simulink model "tutorial40_variant"  (R2025a)
settings: Solver=VariableStepAuto  StartTime=0.0  StopTime=10.0  RelTol=1e-3
settings Model: Creator=xing2  LastModifiedBy=xing2

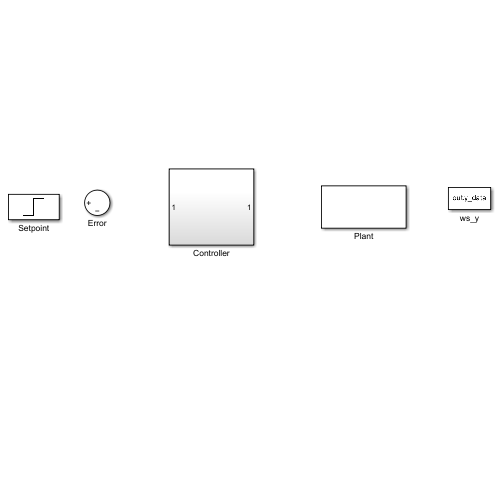
[thumbnail: Simulink's stored preview of the top-level diagram]
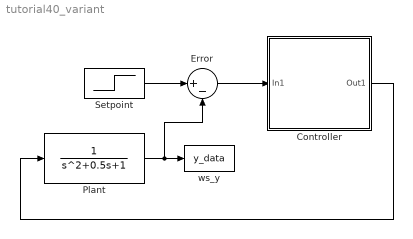
== system tutorial40_variant ==
  Controller : Subsystem  Variant=on
  Error : Sum  Inputs=|+-
  Plant : TransferFcn  Denominator=[1 0.5 1]
  Setpoint : Step  Time=0.5  SampleTime=0
  ws_y : ToWorkspace  VariableName=y_data  SaveFormat=Timeseries  SampleTime=-1
  wires:
  Setpoint/1 -> Error/1
  Plant/1 -> Error/2, ws_y/1
  Error/1 -> Controller/1(In1)
  Controller/1(Out1) -> Plant/1

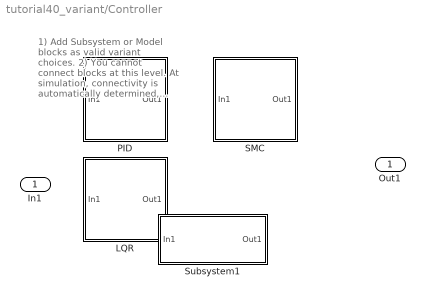
== system tutorial40_variant/Controller ==
  note: 1) Add Subsystem or Model blocks as valid variant choices.
      | 2) You cannot connect blocks at this level. At simulation, connectivity is automatically
      | determined, based on the active variant and port name matching.
  In1 : Inport
  LQR : Subsystem  VariantControl=ctrl_type == 2
  PID : Subsystem  VariantControl=ctrl_type == 1
  SMC : Subsystem  VariantControl=ctrl_type == 3
  Subsystem1 : Subsystem  VariantControl=false
  Out1 : Outport

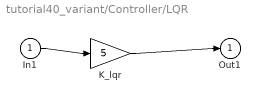
== system tutorial40_variant/Controller/LQR ==
  In1 : Inport
  K_lqr : Gain  Gain=5
  Out1 : Outport
  wires:
  In1/1 -> K_lqr/1
  K_lqr/1 -> Out1/1

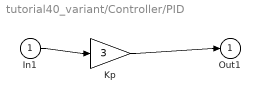
== system tutorial40_variant/Controller/PID ==
  In1 : Inport
  Kp : Gain  Gain=3
  Out1 : Outport
  wires:
  In1/1 -> Kp/1
  Kp/1 -> Out1/1

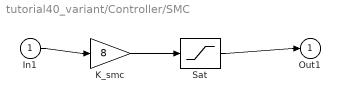
== system tutorial40_variant/Controller/SMC ==
  In1 : Inport
  K_smc : Gain  Gain=8
  Sat : Saturate  UpperLimit=5  LowerLimit=-5
  Out1 : Outport
  wires:
  In1/1 -> K_smc/1
  K_smc/1 -> Sat/1
  Sat/1 -> Out1/1

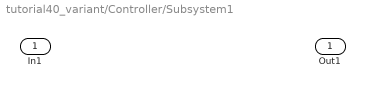
== system tutorial40_variant/Controller/Subsystem1 ==
  In1 : Inport
  Out1 : Outport
